simulink library "sensors_lib"  (Simulink 9.1)
settings: Solver=VariableStepAuto  StartTime=0.0  StopTime=10.0  RelTol=1e-3
undefined symbols (not defined in the file or in its folder): AirData, Vanes
libraries: simulink x9, sensors_S2_lib x2, sensors_T2_lib x1, sensors_T2_design_lib x1, sensors_S2_design_lib x1
settings Model: Creator=amurch  LastModifiedBy=E183308  ExtModeAutoUpdateStatusClock=off

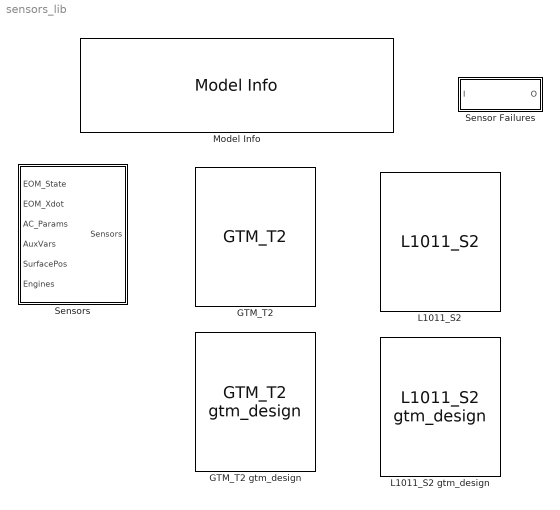
== system sensors_lib ==
  GTM_T2 : sensors_T2_lib/GTM_T2  SystemSampleTime=-1
  GTM_T2 gtm_design : sensors_T2_design_lib/GTM_T2 gtm_design  SystemSampleTime=-1
  L1011_S2 : sensors_S2_lib/L1011_S2  SystemSampleTime=-1
  L1011_S2 gtm_design : sensors_S2_design_lib/L1011_S2 gtm_design  SystemSampleTime=-1
  Model Info : simulink/Model-Wide Utilities/Model Info  Frame=on  DisplayStringWithTags=|  HorizontalTextAlignment=Center  LeftAlignmentValue=0.5
      | Sensor Model Library
      | %<ModelVersion>
      | Las modified by %<LastModifiedBy> on %<LastModificationDate>
  Sensor Failures : Subsystem
  Sensors : Subsystem  BlockChoice=L1011_S2
      settings: TemplateBlock=self  MemberBlocks=GTM_T2,GTM_T2 gtm_design,L1011_S2,L1011_S2 gtm_design

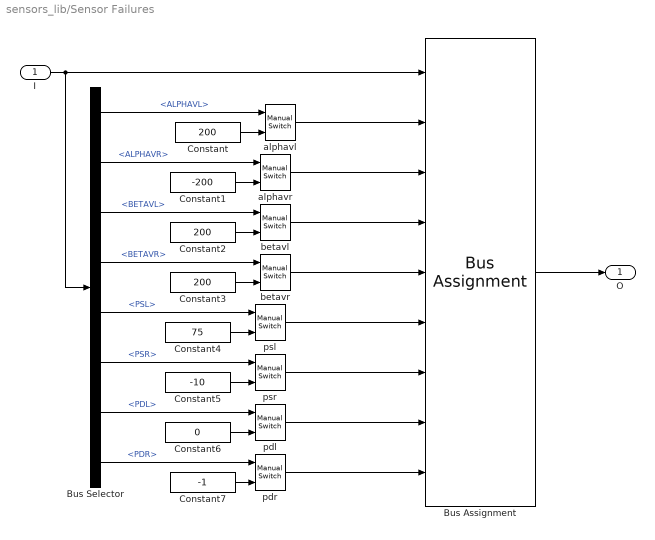
== system sensors_lib/Sensor Failures ==
  I : Inport
  Bus Assignment : BusAssignment  AssignedSignals=Vanes.ALPHAVL,Vanes.ALPHAVR,Vanes.BETAVL,Vanes.BETAVR,AirData.PSL,AirData.PSR,AirData.PDL,AirData.PDR
  Bus Selector : BusSelector  OutputSignals=Vanes.ALPHAVL,Vanes.ALPHAVR,Vanes.BETAVL,Vanes.BETAVR,AirData.PSL,AirData.PSR,AirData.PDL,AirData.PDR
  Constant : Constant  Value=200
  Constant1 : Constant  Value=-200
  Constant2 : Constant  Value=200
  Constant3 : Constant  Value=200
  Constant4 : Constant  Value=75
  Constant5 : Constant  Value=-10
  Constant6 : Constant  Value=0
  Constant7 : Constant  Value=-1
  alphavl : simulink/Signal Routing/Manual Switch  SystemSampleTime=-1  sw=1  action=0  varsize=off
      settings: SourceProductName=Simulink  SourceProductBaseCode=SL
  alphavr : simulink/Signal Routing/Manual Switch  SystemSampleTime=-1  sw=1  action=0  varsize=off
      settings: SourceProductName=Simulink  SourceProductBaseCode=SL
  betavl : simulink/Signal Routing/Manual Switch  SystemSampleTime=-1  sw=1  action=0  varsize=off
      settings: SourceProductName=Simulink  SourceProductBaseCode=SL
  betavr : simulink/Signal Routing/Manual Switch  SystemSampleTime=-1  sw=1  action=0  varsize=off
      settings: SourceProductName=Simulink  SourceProductBaseCode=SL
  pdl : simulink/Signal Routing/Manual Switch  SystemSampleTime=-1  sw=1  action=0  varsize=off
      settings: SourceProductName=Simulink  SourceProductBaseCode=SL
  pdr : simulink/Signal Routing/Manual Switch  SystemSampleTime=-1  sw=1  action=0  varsize=off
      settings: SourceProductName=Simulink  SourceProductBaseCode=SL
  psl : simulink/Signal Routing/Manual Switch  SystemSampleTime=-1  sw=1  action=0  varsize=off
      settings: SourceProductName=Simulink  SourceProductBaseCode=SL
  psr : simulink/Signal Routing/Manual Switch  SystemSampleTime=-1  sw=1  action=0  varsize=off
      settings: SourceProductName=Simulink  SourceProductBaseCode=SL
  O : Outport
  wires:
  I/1 -> Bus Assignment/1, Bus Selector/1
  Bus Assignment/1 -> O/1
  Constant/1 -> alphavl/2
  Bus Selector/1 -> alphavl/1  "<ALPHAVL>"
  alphavl/1 -> Bus Assignment/2
  Constant1/1 -> alphavr/2
  Bus Selector/2 -> alphavr/1  "<ALPHAVR>"
  alphavr/1 -> Bus Assignment/3
  Constant2/1 -> betavl/2
  Bus Selector/3 -> betavl/1  "<BETAVL>"
  betavl/1 -> Bus Assignment/4
  Constant3/1 -> betavr/2
  Bus Selector/4 -> betavr/1  "<BETAVR>"
  betavr/1 -> Bus Assignment/5
  Constant4/1 -> psl/2
  Bus Selector/5 -> psl/1  "<PSL>"
  psl/1 -> Bus Assignment/6
  Constant5/1 -> psr/2
  Bus Selector/6 -> psr/1  "<PSR>"
  psr/1 -> Bus Assignment/7
  Constant6/1 -> pdl/2
  Bus Selector/7 -> pdl/1  "<PDL>"
  pdl/1 -> Bus Assignment/8
  Constant7/1 -> pdr/2
  Bus Selector/8 -> pdr/1  "<PDR>"
  pdr/1 -> Bus Assignment/9

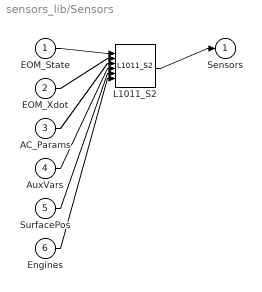
== system sensors_lib/Sensors ==
  EOM_State : Inport
  EOM_Xdot : Inport  Port=2
  AC_Params : Inport  Port=3
  AuxVars : Inport  Port=4
  SurfacePos : Inport  Port=5
  Engines : Inport  Port=6
  L1011_S2 : sensors_S2_lib/L1011_S2  SystemSampleTime=-1
  Sensors : Outport
  wires:
  EOM_State/1 -> L1011_S2/1
  EOM_Xdot/1 -> L1011_S2/2
  AC_Params/1 -> L1011_S2/3
  AuxVars/1 -> L1011_S2/4
  SurfacePos/1 -> L1011_S2/5
  Engines/1 -> L1011_S2/6
  L1011_S2/1 -> Sensors/1
